simulink library "Cal_Loop_Table_lib"  (Simulink 6.6)
undefined symbols (not defined in the file or in its folder): Table, UpCals_Eng, UpCals_Pwm
libraries: simulink x2
settings Model: Creator=cbuttril  LastModifiedBy=cbuttril

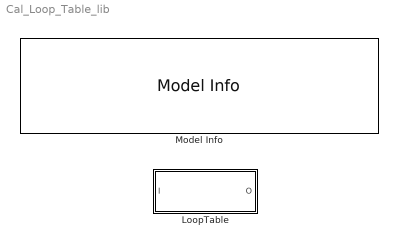
== system Cal_Loop_Table_lib ==
  LoopTable : Subsystem  mask(VectorInterp){XTable=UpCals_Pwm, YTable=UpCals_Eng}
      mask prompts: XTable "Break Point Table"; YTable "Data Value Table"
      mask help:
      | Blocks interpolates multiple input values according to 1-D table lookup.  Each column of Break Point Table and Data Value Table is an independent 1-D mapping.  The vector output represents a 1D lookup on corresponding columns of these tables.
      |
      | Break Point data must be strictly monotonic.
      mask init:
      | % Table lookup requires breakpoint data be strictly monotonically increasing.
      | % Check breakpoint data for a negative slope.
      | badcolumns = find(min(diff(XTable))<=0);
      | 
      | % Try flipping the data over
      | if ~isempty(badcolumns);
      |     for i=badcolumns,
      |         XTable(:,i) = flipud(XTable(:,i));
      |         YTable(:,i) = flipud(YTable(:,i));
      |     end
      | end
      | 
      | % If breakpoing data still has negative slope, it's not monotonic - error out.
      | badcolumns = find(min(diff(XTable))<=0);
      | if ~isempty(badcolumns);
      |     errmsg=sprintf('Break-point data is not monotonic.  Check column(s): ');
      |     errmsg=strcat(errmsg,sprintf(' %d ',badcolumns));
      |     error(errmsg);
      | end
  Model Info : simulink/Model-Wide Utilities/Model Info  SystemSampleTime=-1  InitialBlockCM=None  BlockCM=None  Frame=on  DisplayStringWithTags=|  HorizontalTextAlignment=Center  LeftAlignmentValue=0.5  SourceBlockDiagram=Cal_Loop_Table_lib  TagMaxNumber=20
      | Developed using Matlab Release 2007a
      | 
      | SVN:%<ModelVersion>
      | Last modifed by %<LastModifiedBy> on %<LastModificationDate>

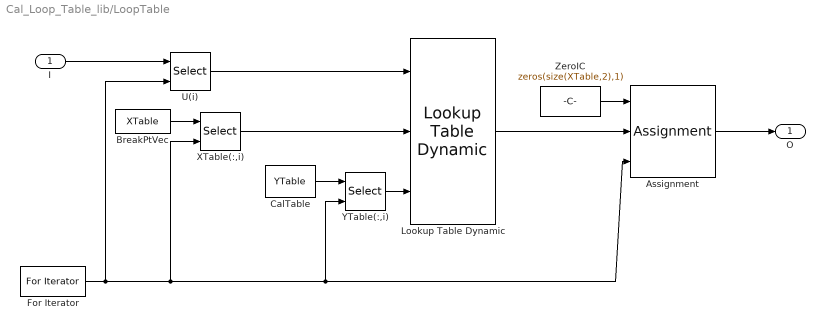
== system Cal_Loop_Table_lib/LoopTable ==
  I : Inport
  Assignment : Assignment  IndexMode=Zero-based  IndexOptions=Index vector (port)  Indices=1  OutputSizes=1
  BreakPtVec : Constant  Value=XTable
  CalTable : Constant  Value=YTable
  For Iterator : ForIterator  IterationLimit=size(XTable,2)  IndexMode=Zero-based
  Lookup Table Dynamic : simulink/Lookup Tables/Lookup Table Dynamic  LookUpMeth=Interpolation-Use End Values  OutputDataTypeScalingMode=Specify via dialog  OutDataType=float('double')  OutScaling=2^-10  DoSatur=off
  U(i) : Selector  IndexMode=Zero-based  IndexOptions=Index vector (port)  Indices=[1 3]  OutputSizes=1  InputPortWidth=size(XTable,2)
  XTable(:,i) : Selector  NumberOfDimensions=2  IndexMode=Zero-based  IndexOptions=Select all,Index vector (port)  Indices=[1 3],1  OutputSizes=1,1  InputPortWidth=size(Table,2)
  YTable(:,i) : Selector  NumberOfDimensions=2  IndexMode=Zero-based  IndexOptions=Select all,Index vector (port)  Indices=[1 3],1  OutputSizes=1,1  InputPortWidth=size(Table,2)
  ZeroIC : Constant  Value=zeros(size(XTable,2),1)
  O : Outport
  wires:
  XTable(:,i)/1 -> Lookup Table Dynamic/2
  BreakPtVec/1 -> XTable(:,i)/1
  YTable(:,i)/1 -> Lookup Table Dynamic/3
  CalTable/1 -> YTable(:,i)/1
  U(i)/1 -> Lookup Table Dynamic/1
  I/1 -> U(i)/1
  Lookup Table Dynamic/1 -> Assignment/2
  Assignment/1 -> O/1
  ZeroIC/1 -> Assignment/1
  For Iterator/1 -> XTable(:,i)/2, Assignment/3, YTable(:,i)/2, U(i)/2
